simulink library "INT_AFST_DD"  (R2016b)
settings: Solver=VariableStepAuto  StartTime=0.0  StopTime=10.0  RelTol=1e-3
settings Model: Creator=guanxiaoxing  LastModifiedBy=guanxiaoxing

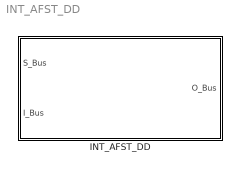
== system INT_AFST_DD ==
  INT_AFST_DD : Subsystem

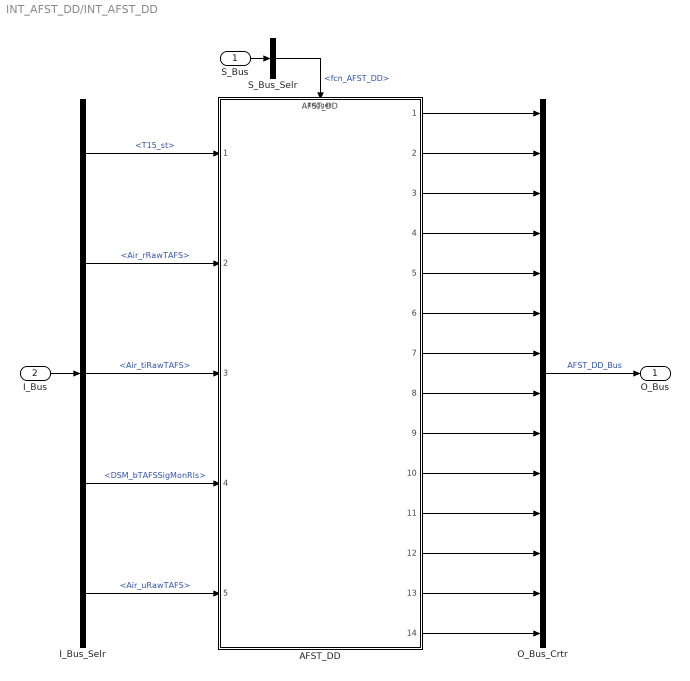
== system INT_AFST_DD/INT_AFST_DD ==
  S_Bus : Inport
  I_Bus : Inport  Port=2
  AFST_DD : ModelReference  ModelNameDialog=AFST_DD  SimulationMode=Normal  ModelReferenceVersion=1.46  TriggerPortName=function  TriggerPortTriggerType=function-call  TriggerPortStatesWhenEnabling=held
  I_Bus_Selr : BusSelector  OutputSignals=T15_st,Air_rRawTAFS,Air_tiRawTAFS,DSM_bTAFSSigMonRls,Air_uRawTAFS
  O_Bus_Crtr : BusCreator  Inputs=14
  S_Bus_Selr : BusSelector  OutputSignals=fcn_AFST_DD
  O_Bus : Outport
  wires:
  S_Bus_Selr/1 -> AFST_DD/Trigger  "<fcn_AFST_DD>"
  S_Bus/1 -> S_Bus_Selr/1
  I_Bus/1 -> I_Bus_Selr/1
  I_Bus_Selr/1 -> AFST_DD/1  "<T15_st>"
  I_Bus_Selr/2 -> AFST_DD/2  "<Air_rRawTAFS>"
  I_Bus_Selr/3 -> AFST_DD/3  "<Air_tiRawTAFS>"
  I_Bus_Selr/4 -> AFST_DD/4  "<DSM_bTAFSSigMonRls>"
  I_Bus_Selr/5 -> AFST_DD/5  "<Air_uRawTAFS>"
  O_Bus_Crtr/1 -> O_Bus/1  "AFST_DD_Bus"
  AFST_DD/1 -> O_Bus_Crtr/1
  AFST_DD/2 -> O_Bus_Crtr/2
  AFST_DD/3 -> O_Bus_Crtr/3
  AFST_DD/4 -> O_Bus_Crtr/4
  AFST_DD/5 -> O_Bus_Crtr/5
  AFST_DD/6 -> O_Bus_Crtr/6
  AFST_DD/7 -> O_Bus_Crtr/7
  AFST_DD/8 -> O_Bus_Crtr/8
  AFST_DD/9 -> O_Bus_Crtr/9
  AFST_DD/10 -> O_Bus_Crtr/10
  AFST_DD/11 -> O_Bus_Crtr/11
  AFST_DD/12 -> O_Bus_Crtr/12
  AFST_DD/13 -> O_Bus_Crtr/13
  AFST_DD/14 -> O_Bus_Crtr/14
